simulink model "main"  (Simulink 3.00)
undefined symbols (not defined in the file): geas
libraries: genlib x2, matrixlib x1, mathlib x1, arclib x1

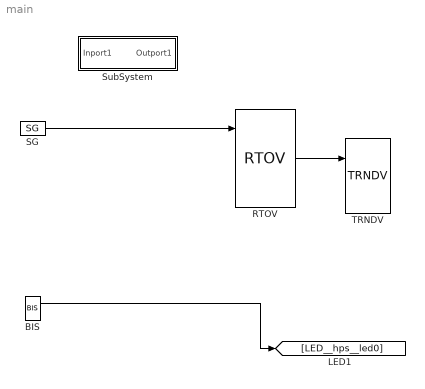
== system main ==
  BIS : genlib/BIS  Y0=off  t1=0.2  t2=0.4  t3=0.0000000E+000  t4=4.0000000E+000  t5=5.0000000E+000  t6=6.0000000E+000  t7=7.0000000E+000  t8=8.0000000E+000  RPT=on
  RTOV : matrixlib/RTOV  capacity=8  offset=0  n=8  Type=8: Double
  SG : genlib/SG  isig=1: SINE  amp=1.0000000E+000  freq=1.0000000E+000  phase=0.0000000E+000  ifrunit=1: Hz  iphunit=1: degrees
  SubSystem : Subsystem  mask(REX sequence){Par1=geas}
      mask prompts: Par1 "sdaghrst"
  TRNDV : arclib/TRNDV  n=8  l=1000  btype=8: Double  pfac=1  afac=0  arc=0  id=1  Title=Trend Title
  wires:
  BIS/1 -> [LED__hps__led0]
  ? -> RTOV/3
  ? -> RTOV/4
  RTOV/1 -> TRNDV/1
  SG/1 -> RTOV/2

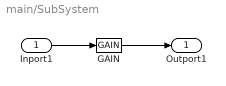
== system main/SubSystem ==
  Inport1 : Inport  Port=1
  GAIN : mathlib/GAIN  k=1
  Outport1 : Outport  Port=1
  wires:
  GAIN/1 -> Outport1/1
  Inport1/1 -> GAIN/1
